simulink model "model_euler"  (R2018b)
settings: Solver=VariableStepAuto  StartTime=0.0  StopTime=10  RelTol=1e-3
settings Model: Creator=SHRUTI  LastModifiedBy=SHRUTI

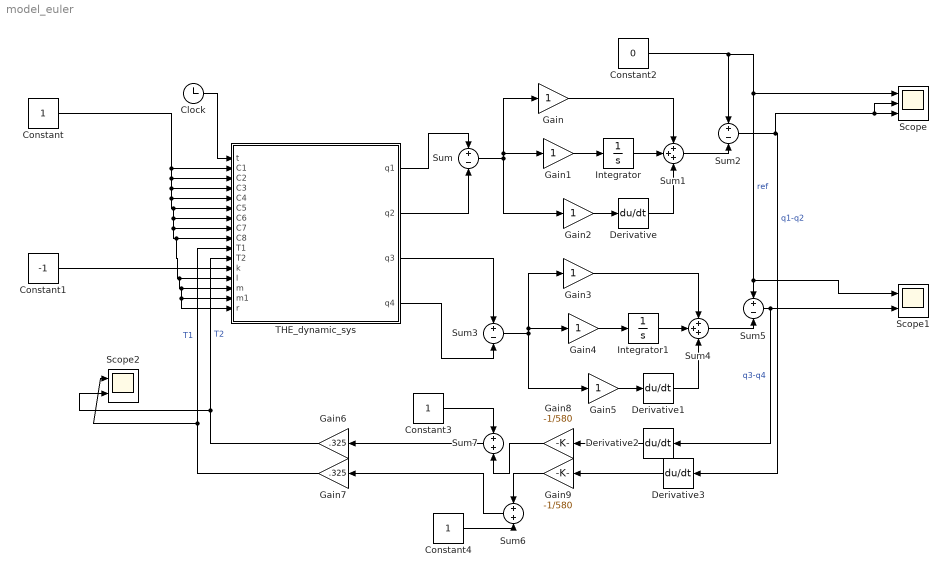
== system model_euler ==
  Clock : Clock
  Constant : Constant
  Constant1 : Constant  Value=-1
  Constant2 : Constant  Value=0
  Constant3 : Constant
  Constant4 : Constant
  Derivative{,1..3} (4 alike) : Derivative
  Gain{,1..5} (6 alike) : Gain
  Gain6 : Gain  Gain=.325
  Gain7 : Gain  Gain=.325
  Gain8 : Gain  Gain=-1/580
  Gain9 : Gain  Gain=-1/580
  Integrator : Integrator
  Integrator1 : Integrator
  Scope : Scope  NumInputPorts=3
  Scope1 : Scope  NumInputPorts=2
  Scope2 : Scope  NumInputPorts=2
  Sum{,2..3,5} (4 alike) : Sum  Inputs=+-
  Sum1 : Sum  Inputs=+++
  Sum4 : Sum  Inputs=+++
  Sum6 : Sum
  Sum7 : Sum
  THE_dynamic_sys : MATLAB Function  TreatAsAtomicUnit=on
  wires:
  Constant/1 -> THE_dynamic_sys/15(m1), THE_dynamic_sys/16(r), THE_dynamic_sys/14(m), THE_dynamic_sys/13(l), THE_dynamic_sys/9(C8), THE_dynamic_sys/8(C7), THE_dynamic_sys/7(C6), THE_dynamic_sys/6(C5), THE_dynamic_sys/5(C4), THE_dynamic_sys/4(C3), THE_dynamic_sys/3(C2), THE_dynamic_sys/2(C1)
  Constant1/1 -> THE_dynamic_sys/12(k)
  Clock/1 -> THE_dynamic_sys/1(t)
  THE_dynamic_sys/1(q1) -> Sum/1
  THE_dynamic_sys/2(q2) -> Sum/2
  Sum/1 -> Gain2/1, Gain1/1, Gain/1
  Gain2/1 -> Derivative/1
  Gain1/1 -> Integrator/1
  Integrator/1 -> Sum1/2
  Gain/1 -> Sum1/1
  Derivative/1 -> Sum1/3
  Constant2/1 -> Scope/1, Scope1/1, Sum5/1, Sum2/1  "ref"
  Sum1/1 -> Sum2/2
  Sum3/1 -> Gain5/1, Gain4/1, Gain3/1
  Integrator1/1 -> Sum4/2
  Sum4/1 -> Sum5/2
  Gain4/1 -> Integrator1/1
  Gain5/1 -> Derivative1/1
  Derivative1/1 -> Sum4/3
  THE_dynamic_sys/3(q3) -> Sum3/1
  THE_dynamic_sys/4(q4) -> Sum3/2
  Gain3/1 -> Sum4/1
  Sum2/1 -> Scope/2, Scope/3, Derivative3/1  "q1-q2"
  Sum5/1 -> Derivative2/1, Scope1/2  "q3-q4"
  Gain6/1 -> Scope2/2, THE_dynamic_sys/11(T2)  "T2"
  Gain7/1 -> Scope2/1, THE_dynamic_sys/10(T1)  "T1"
  Constant4/1 -> Sum6/2
  Gain9/1 -> Sum6/1
  Sum6/1 -> Gain7/1
  Sum7/1 -> Gain6/1
  Gain8/1 -> Sum7/2
  Constant3/1 -> Sum7/1
  Derivative2/1 -> Gain8/1
  Derivative3/1 -> Gain9/1

== matlab function model_euler/THE_dynamic_sys ==
  data: t input; q1 output; C1 input; C2 input; C3 input; C4 input; C5 input; C6 input; C7 input; C8 input; T1 input; T2 input; k input; l input; m input; m1 input; r input; q2 output; q3 output; q4 output
function [q1,q2,q3,q4] = THE_dynamic_sys(t,C1,C2,C3,C4,C5,C6,C7,C8,T1,T2,k,l,m,m1,r)
%#codegen

%    This function was generated by the Symbolic Math Toolbox version 8.2.
%    13-Jan-2019 20:54:21

q1 = (l.^2.*m.*(C1-(T1.*1.0./l.^2.*m1.*r.^2.*t.^2)./(m.*2.0)))./(l.^2.*m+m1.*r.^2)+(l.^2.*m.*t.*(C3+(T1.*1.0./l.^2.*m1.*r.^2.*t)./m))./(l.^2.*m+m1.*r.^2)+(sqrt(2.0).*1.0./sqrt(-k).*l.^5.*m.^(5.0./2.0).*1.0./sqrt(m1).*exp((sqrt(2.0).*sqrt(-k).*1.0./sqrt(m).*1.0./sqrt(m1).*t.*sqrt(l.^2.*m+m1.*r.^2))./(l.*r)).*1.0./(l.^2.*m+m1.*r.^2).^(3.0./2.0).*(C5-(sqrt(2.0).*T1.*1.0./sqrt(-k).*1.0./sqrt(m).*m1.^(3.0./2.0).*r.^3.*exp(-(sqrt(2.0).*sqrt(-k).*1.0./sqrt(m).*1.0./sqrt(m1).*t.*sqrt(l.^2.*m+m1.*r.^2))./(l.*r)).*1.0./sqrt(l.^2.*m+m1.*r.^2))./(l.*2.0)))./(r.*4.0)-(sqrt(2.0).*1.0./sqrt(-k).*l.^5.*m.^(5.0./2.0).*1.0./sqrt(m1).*exp(-(sqrt(2.0).*sqrt(-k).*1.0./sqrt(m).*1.0./sqrt(m1).*t.*sqrt(l.^2.*m+m1.*r.^2))./(l.*r)).*1.0./(l.^2.*m+m1.*r.^2).^(3.0./2.0).*(C6+(sqrt(2.0).*T1.*1.0./sqrt(-k).*1.0./sqrt(m).*m1.^(3.0./2.0).*r.^3.*exp((sqrt(2.0).*sqrt(-k).*1.0./sqrt(m).*1.0./sqrt(m1).*t.*sqrt(l.^2.*m+m1.*r.^2))./(l.*r)).*1.0./sqrt(l.^2.*m+m1.*r.^2))./(l.*2.0)))./(r.*4.0);
if nargout > 1
    q2 = (l.^2.*m.*(C1-(T1.*1.0./l.^2.*m1.*r.^2.*t.^2)./(m.*2.0)))./(l.^2.*m+m1.*r.^2)+(l.^2.*m.*t.*(C3+(T1.*1.0./l.^2.*m1.*r.^2.*t)./m))./(l.^2.*m+m1.*r.^2)-(sqrt(2.0).*1.0./sqrt(-k).*l.^3.*m.^(3.0./2.0).*sqrt(m1).*r.*exp((sqrt(2.0).*sqrt(-k).*1.0./sqrt(m).*1.0./sqrt(m1).*t.*sqrt(l.^2.*m+m1.*r.^2))./(l.*r)).*1.0./(l.^2.*m+m1.*r.^2).^(3.0./2.0).*(C5-(sqrt(2.0).*T1.*1.0./sqrt(-k).*1.0./sqrt(m).*m1.^(3.0./2.0).*r.^3.*exp(-(sqrt(2.0).*sqrt(-k).*1.0./sqrt(m).*1.0./sqrt(m1).*t.*sqrt(l.^2.*m+m1.*r.^2))./(l.*r)).*1.0./sqrt(l.^2.*m+m1.*r.^2))./(l.*2.0)))./4.0+(sqrt(2.0).*1.0./sqrt(-k).*l.^3.*m.^(3.0./2.0).*sqrt(m1).*r.*exp(-(sqrt(2.0).*sqrt(-k).*1.0./sqrt(m).*1.0./sqrt(m1).*t.*sqrt(l.^2.*m+m1.*r.^2))./(l.*r)).*1.0./(l.^2.*m+m1.*r.^2).^(3.0./2.0).*(C6+(sqrt(2.0).*T1.*1.0./sqrt(-k).*1.0./sqrt(m).*m1.^(3.0./2.0).*r.^3.*exp((sqrt(2.0).*sqrt(-k).*1.0./sqrt(m).*1.0./sqrt(m1).*t.*sqrt(l.^2.*m+m1.*r.^2))./(l.*r)).*1.0./sqrt(l.^2.*m+m1.*r.^2))./(l.*2.0)))./4.0;
end
if nargout > 2
    q3 = (l.^2.*m.*(C2-(T2.*1.0./l.^2.*m1.*r.^2.*t.^2)./(m.*2.0)))./(l.^2.*m+m1.*r.^2)+(l.^2.*m.*t.*(C4+(T2.*1.0./l.^2.*m1.*r.^2.*t)./m))./(l.^2.*m+m1.*r.^2)+(sqrt(2.0).*1.0./sqrt(-k).*l.^5.*m.^(5.0./2.0).*1.0./sqrt(m1).*exp((sqrt(2.0).*sqrt(-k).*1.0./sqrt(m).*1.0./sqrt(m1).*t.*sqrt(l.^2.*m+m1.*r.^2))./(l.*r)).*1.0./(l.^2.*m+m1.*r.^2).^(3.0./2.0).*(C7-(sqrt(2.0).*T2.*1.0./sqrt(-k).*1.0./sqrt(m).*m1.^(3.0./2.0).*r.^3.*exp(-(sqrt(2.0).*sqrt(-k).*1.0./sqrt(m).*1.0./sqrt(m1).*t.*sqrt(l.^2.*m+m1.*r.^2))./(l.*r)).*1.0./sqrt(l.^2.*m+m1.*r.^2))./(l.*2.0)))./(r.*4.0)-(sqrt(2.0).*1.0./sqrt(-k).*l.^5.*m.^(5.0./2.0).*1.0./sqrt(m1).*exp(-(sqrt(2.0).*sqrt(-k).*1.0./sqrt(m).*1.0./sqrt(m1).*t.*sqrt(l.^2.*m+m1.*r.^2))./(l.*r)).*1.0./(l.^2.*m+m1.*r.^2).^(3.0./2.0).*(C8+(sqrt(2.0).*T2.*1.0./sqrt(-k).*1.0./sqrt(m).*m1.^(3.0./2.0).*r.^3.*exp((sqrt(2.0).*sqrt(-k).*1.0./sqrt(m).*1.0./sqrt(m1).*t.*sqrt(l.^2.*m+m1.*r.^2))./(l.*r)).*1.0./sqrt(l.^2.*m+m1.*r.^2))./(l.*2.0)))./(r.*4.0);
end
if nargout > 3
    q4 = (l.^2.*m.*(C2-(T2.*1.0./l.^2.*m1.*r.^2.*t.^2)./(m.*2.0)))./(l.^2.*m+m1.*r.^2)+(l.^2.*m.*t.*(C4+(T2.*1.0./l.^2.*m1.*r.^2.*t)./m))./(l.^2.*m+m1.*r.^2)-(sqrt(2.0).*1.0./sqrt(-k).*l.^3.*m.^(3.0./2.0).*sqrt(m1).*r.*exp((sqrt(2.0).*sqrt(-k).*1.0./sqrt(m).*1.0./sqrt(m1).*t.*sqrt(l.^2.*m+m1.*r.^2))./(l.*r)).*1.0./(l.^2.*m+m1.*r.^2).^(3.0./2.0).*(C7-(sqrt(2.0).*T2.*1.0./sqrt(-k).*1.0./sqrt(m).*m1.^(3.0./2.0).*r.^3.*exp(-(sqrt(2.0).*sqrt(-k).*1.0./sqrt(m).*1.0./sqrt(m1).*t.*sqrt(l.^2.*m+m1.*r.^2))./(l.*r)).*1.0./sqrt(l.^2.*m+m1.*r.^2))./(l.*2.0)))./4.0+(sqrt(2.0).*1.0./sqrt(-k).*l.^3.*m.^(3.0./2.0).*sqrt(m1).*r.*exp(-(sqrt(2.0).*sqrt(-k).*1.0./sqrt(m).*1.0./sqrt(m1).*t.*sqrt(l.^2.*m+m1.*r.^2))./(l.*r)).*1.0./(l.^2.*m+m1.*r.^2).^(3.0./2.0).*(C8+(sqrt(2.0).*T2.*1.0./sqrt(-k).*1.0./sqrt(m).*m1.^(3.0./2.0).*r.^3.*exp((sqrt(2.0).*sqrt(-k).*1.0./sqrt(m).*1.0./sqrt(m1).*t.*sqrt(l.^2.*m+m1.*r.^2))./(l.*r)).*1.0./sqrt(l.^2.*m+m1.*r.^2))./(l.*2.0)))./4.0;
end
